simulink model "SIM_6DOF_completo_qnathy_comparaPeixoto"  (R2021b)
settings: Solver=FixedStepAuto  StartTime=0.0  StopTime=D.Tfim  FixedStep=0.001  MaxStep=0.001  RelTol=1e-3
undefined symbols (not defined in the file or in its folder): c, D, dados, desv_emp, erro, F, Light, M, MIL, Newton, Raphson, wind
libraries: aerolibasang x7, sharedutil x3, aerolibwind2 x3, shared6dof x2, aerolibanim x1, aerolibatmos2 x1, simulink x1, dspmtrx3 x1, sharedtransform x1
(part 2 of 2)

== system SIM_6DOF_completo_qnathy_comparaPeixoto/Dinamica 6DOF/Aerodinamica/Subsystem8/Subsystem6 ==
  d : Inport
  Velocity : Inport  Port=2
  Divide : Product  Inputs=*/
  d/(2V) : Gain  Gain=1/2  SaturateOnIntegerOverflow=on  OutDataTypeStr=Inherit: Same as input  ParamDataTypeStr=Inherit: Same as input
  dot : aerolibasang/Dynamic Pressure/dot  SystemSampleTime=-1  VariantActivationTime=update diagram  Latency=0  AutoFrameSizeCalculation=off
      settings: SourceProductBaseCode=AE
  vt : Sqrt  AlgorithmType=Newton-Raphson  SaturateOnIntegerOverflow=on
  d2V : Outport  InitialOutput=0  VectorParamsAs1DForOutWhenUnconnected=off
  wires:
  d/(2V)/1 -> d2V/1
  Velocity/1 -> dot/1
  Divide/1 -> d/(2V)/1
  dot/1 -> vt/1
  d/1 -> Divide/1
  vt/1 -> Divide/2
